simulink model "QCwithActDyn_NewPID"  (R2020a)
settings: Solver=FixedStepAuto  StartTime=0.0  StopTime=5+T  FixedStep=0.001  RelTol=1e-3
model workspace (MAT data in the model file):
  time_step = 0.01
values from neighbouring files (symbols this model uses):
  K_pitch = 30    [Parameters.m]
  K_roll = 30    [Parameters.m]
  K_z = 1.5059    [Parameters.m]    (also in descent2.m = 2)
  kD_P = 0.1529    [Parameters.m]
  kD_R = 0.1564    [Parameters.m]
  kD_x = 9.3766    [Parameters.m]
  kD_y = 9.54    [Parameters.m]
  kD_z = 17    [Parameters.m]    (also in descent2.m = 17.85; gradient_descent.m = 0.95*kD_z)
  kI_x = 0    [Parameters.m]
  kI_y = 0    [Parameters.m]
  kP_P = 1.3542    [Parameters.m]
  kP_R = 1.3852    [Parameters.m]
  kP_x = 34.159    [Parameters.m]
  kP_y = 34.775    [Parameters.m]
  kP_z = 40    [Parameters.m]    (also in descent2.m; gradient_descent.m = 0.95*kP_z)
  PVA = 1    [Parameters.m]
  T_aero = 1.5    [Parameters.m]    (also in descent2.m = 2)
  T_motor = 0.015    [Parameters.m]
  T_pitch = 0.2005    [Parameters.m]
  tau_pitch = 0.025    [Parameters.m]
  tau_roll = 0.025    [Parameters.m]
  tau_x = 0.0223    [Parameters.m]
  tau_y = 0.0223    [Parameters.m]
  tau_z = 0.027    [Parameters.m]
  X_Ch = 1    [Parameters.m]
  Y_Ch = 1    [Parameters.m]
libraries: simulink_extras x2
settings Model: Creator=Abdulaziz Y. Alkayas  LastModifiedBy=anees
settings SolverCC: SolverResetMethod=Robust
settings DebuggingCC: UnconnectedInputMsg=none  UnconnectedOutputMsg=none  ArithmeticOperatorsInVariantConditions=warning
settings HardwareCC: TargetBitPerPointer=64  TargetBitPerSizeT=64  TargetBitPerPtrDiffT=64  TargetLongLongMode=on  TargetIntDivRoundTo=Zero  TargetEndianess=LittleEndian  TargetWordSize=64  TargetHWDeviceType=MATLAB Host  ProdEqTarget=off
settings SFSimCC: CustomCodeUndefinedFunction=UseInterfaceOnly
settings RTWCC: Description=Generic Real-Time Target

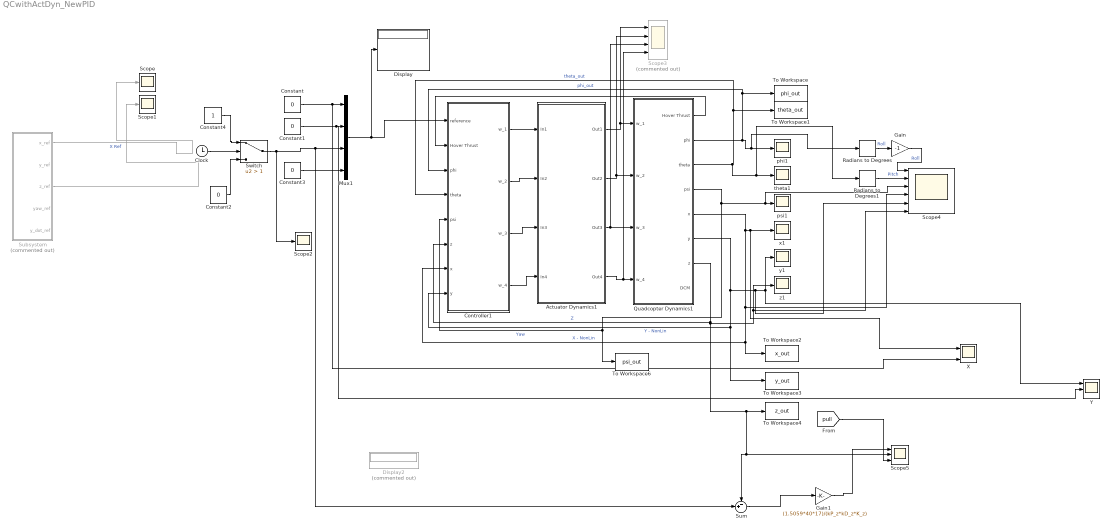
== system QCwithActDyn_NewPID ==
  Actuator Dynamics1 : Subsystem
  Clock : Clock
  Constant{,1..3} (4 alike) : Constant  Value=0
  Constant4 : Constant
  Controller1 : Subsystem
  Display : Display
  Display2 : Display  Commented=on
  Gain : Gain  Gain=-1
  Gain1 : Gain  Gain=(1.5059*40*17)/(kP_z*kD_z*K_z)
  Mux1 : Mux
  Quadcopter Dynamics1 : Subsystem
  Radians to Degrees : simulink_extras/Transformations/Radians to Degrees
  Radians to Degrees1 : simulink_extras/Transformations/Radians to Degrees
  Scope : Scope
  Scope1 : Scope
  Scope2 : Scope
  Scope3 : Scope  Commented=on  NumInputPorts=4
  Scope4 : Scope  NumInputPorts=6
  Scope5 : Scope  NumInputPorts=3
  Subsystem : Subsystem  Commented=on
  Sum : Sum  Inputs=-+|
  Switch : Switch  Criteria=u2 > Threshold  Threshold=1
  To Workspace : ToWorkspace  VariableName=phi_out  SaveFormat=Timeseries  SampleTime=-1
  To Workspace1 : ToWorkspace  VariableName=theta_out  SaveFormat=Timeseries  SampleTime=-1
  To Workspace2 : ToWorkspace  VariableName=x_out  SaveFormat=Timeseries  SampleTime=-1
  To Workspace3 : ToWorkspace  VariableName=y_out  SaveFormat=Timeseries  SampleTime=-1
  To Workspace4 : ToWorkspace  VariableName=z_out  SaveFormat=Timeseries  SampleTime=-1
  To Workspace6 : ToWorkspace  VariableName=psi_out  SaveFormat=Timeseries  SampleTime=-1
  X : Scope  NumInputPorts=3
  Y : Scope  NumInputPorts=3
  phi1 : Scope
  psi1 : Scope
  theta1 : Scope
  x1 : Scope
  y1 : Scope
  z1 : Scope
  wires:
  Controller1/4(w_4) -> Actuator Dynamics1/4(In4)
  Controller1/3(w_3) -> Actuator Dynamics1/3(In3)
  Controller1/2(w_2) -> Actuator Dynamics1/2(In2)
  Controller1/1(w_1) -> Actuator Dynamics1/1(In1)
  Quadcopter Dynamics1/4(psi) -> To Workspace6/1, Controller1/5(psi), psi1/1, Scope4/3  "Yaw"
  Quadcopter Dynamics1/7(z) -> Sum/1, Scope5/2, To Workspace4/1, z1/1, Scope4/6, Controller1/6(z)  "Z"
  Quadcopter Dynamics1/1(Hover Thrust) -> Controller1/2(Hover Thrust)
  Quadcopter Dynamics1/5(x) -> Scope4/4, To Workspace2/1, Controller1/7(x), X/1, x1/1  "X - NonLin"
  Quadcopter Dynamics1/6(y) -> To Workspace3/1, Controller1/8(y), Y/1, y1/1, Scope4/5  "Y - NonLin"
  Subsystem/3("z_ref ") -> Scope1/1
  Actuator Dynamics1/1(Out1) -> Scope3/1, Quadcopter Dynamics1/1(w_1)
  Actuator Dynamics1/2(Out2) -> Quadcopter Dynamics1/2(w_2), Scope3/2
  Actuator Dynamics1/3(Out3) -> Quadcopter Dynamics1/3(w_3), Scope3/3
  Actuator Dynamics1/4(Out4) -> Quadcopter Dynamics1/4(w_4), Scope3/4
  Radians to Degrees/1 -> Gain/1  "Roll"
  Radians to Degrees1/1 -> Scope4/2  "Pitch"
  Gain/1 -> Scope4/1  "Roll"
  Subsystem/1("x_ref ") -> Scope/1  "X Ref"
  Constant1/1 -> Y/2, Mux1/2
  Constant/1 -> X/3, Mux1/1
  Constant3/1 -> Mux1/4
  Mux1/1 -> Display/1, Controller1/1(reference)
  Quadcopter Dynamics1/2(phi) -> Controller1/3(phi), To Workspace/1, Radians to Degrees/1, phi1/1  "phi_out"
  Quadcopter Dynamics1/3(theta) -> Radians to Degrees1/1, theta1/1, Controller1/4(theta), To Workspace1/1  "theta_out"
  Constant2/1 -> Switch/3
  Switch/1 -> Sum/2, Mux1/3, Scope2/1
  Constant4/1 -> Switch/1
  Clock/1 -> Switch/2
  [pull] -> Scope5/3
  Gain1/1 -> Scope5/1
  Sum/1 -> Gain1/1

== system QCwithActDyn_NewPID/Actuator Dynamics1 ==
  In1 : Inport
  In2 : Inport  Port=2
  In3 : Inport  Port=3
  In4 : Inport  Port=4
  Transfer Fcn{1..4} (4 alike) : TransferFcn  Denominator=[T_motor 1]
  Out1 : Outport
  Out2 : Outport  Port=2
  Out3 : Outport  Port=3
  Out4 : Outport  Port=4
  wires:
  In4/1 -> Transfer Fcn2/1
  Transfer Fcn2/1 -> Out4/1
  Transfer Fcn1/1 -> Out3/1
  In2/1 -> Transfer Fcn4/1
  Transfer Fcn4/1 -> Out2/1
  Transfer Fcn3/1 -> Out1/1
  In3/1 -> Transfer Fcn1/1
  In1/1 -> Transfer Fcn3/1

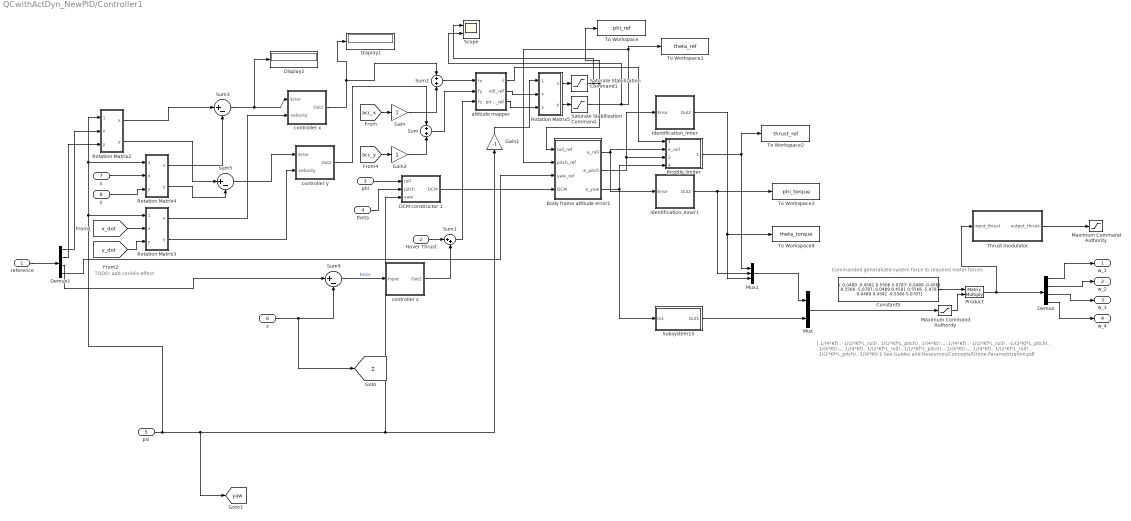
== system QCwithActDyn_NewPID/Controller1 ==
  note: TODO: add coriolis effect
  note: [ 1/(4*Kf) , -1/(2*Kf*L_roll) , 1/(2*Kf*L_pitch) , 1/(4*Kt) ;...
      | 1/(4*Kf) , -1/(2*Kf*L_roll) , -1/(2*Kf*L_pitch) , -1/(4*Kt) ;...
      | 1/(4*Kf) , 1/(2*Kf*L_roll) , 1/(2*Kf*L_pitch) , -1/(4*Kt) ;...
      | 1/(4*Kf) , 1/(2*Kf*L_roll) , -1/(2*Kf*L_pitch) , 1/(4*Kt) ];
      |
      | See Guides and Resources/Concepts/Drone Parametrization.pdf
  note: Commanded generalized system force to required motor forces
  reference : Inport
  Hover Thrust : Inport  Port=2
  phi : Inport  Port=3
  theta : Inport  Port=4
  psi : Inport  Port=5
  z : Inport  Port=6
  x : Inport  Port=7
  y : Inport  Port=8
  Body frame attitude error1 : MATLAB Function  TreatAsAtomicUnit=on
  Constant5 : Constant  Value=|
      | [ 0.0489   -0.4581    0.5566    5.0787;
      |   0.0489   -0.4581   -0.5566   -5.0787;
      |   0.0489    0.4581    0.5566   -5.0787;
      |   0.0489    0.4581   -0.5566    5.0787]
  DCM constructor 1 : MATLAB Function  TreatAsAtomicUnit=on
  Demux : Demux
  Demux1 : Demux
  Display1 : Display
  Display2 : Display
  Gain : Gain
  Gain1 : Gain  Gain=-1
  Gain2 : Gain
  Identification_Inner : Subsystem
  Identification_Inner1 : Subsystem
  Maximum Command Authority : Saturate  UpperLimit=[Inf Inf Inf Inf]  LowerLimit=[-inf -Inf -Inf -Inf]
  "Maximum Command Authority " : Saturate  UpperLimit=[1 1 1 1]  LowerLimit=[0 0 0 0]
  Mux : Mux  Inputs=[3, 1]
  Mux1 : Mux  Inputs=3
  Product : Product  Multiplication=Matrix(*)
  Rotation Matrix2 : Subsystem
  Rotation Matrix3 : Subsystem
  Rotation Matrix4 : Subsystem
  Rotation Matrix5 : Subsystem
  Saturate Stabilization Command : Saturate  UpperLimit=pi/2  LowerLimit=-pi/2
  Saturate Stabilization Command1 : Saturate  UpperLimit=pi/2  LowerLimit=-pi/2
  Scope : Scope  NumInputPorts=2
  Subsystem15 : Subsystem
  Sum : Sum
  Sum1 : Sum  Inputs=|++
  Sum2 : Sum
  Sum3 : Sum  Inputs=|+-
  Sum5 : Sum  Inputs=|+-
  Sum9 : Sum  Inputs=|+-
  Thrust modulator : MATLAB Function  TreatAsAtomicUnit=on
  To Workspace : ToWorkspace  VariableName=phi_ref  SaveFormat=Structure With Time  SampleTime=-1
  To Workspace1 : ToWorkspace  VariableName=theta_ref  SaveFormat=Structure With Time  SampleTime=-1
  To Workspace2 : ToWorkspace  VariableName=thrust_ref  SaveFormat=Timeseries  SampleTime=-1
  To Workspace3 : ToWorkspace  VariableName=phi_torque  SaveFormat=Timeseries  SampleTime=-1
  To Workspace4 : ToWorkspace  VariableName=theta_torque  SaveFormat=Timeseries  SampleTime=-1
  "attitude mapper " : MATLAB Function  TreatAsAtomicUnit=on
  controller x : Subsystem
  controller y : Subsystem
  controller z : Subsystem
  throttle limiter : MATLAB Function  TreatAsAtomicUnit=on
  w_1 : Outport
  w_2 : Outport  Port=2
  w_3 : Outport  Port=3
  w_4 : Outport  Port=4
  tag scope: yaw=global, z=global
  wires:
  z/1 -> Sum9/2, [z]
  Maximum Command Authority/1 -> Product/2
  Mux/1 -> Maximum Command Authority/1
  Constant5/1 -> Product/1
  Demux/2 -> w_2/1
  Demux/3 -> w_3/1
  Demux/4 -> w_4/1
  Sum3/1 -> Display2/1, controller x/1(Error)
  Sum5/1 -> controller y/1(Error)
  Hover Thrust/1 -> Sum1/1
  Demux/1 -> w_1/1
  Sum9/1 -> controller z/1(Input)  "Error"
  controller z/1(Out2) -> Sum1/2
  reference/1 -> Demux1/1
  Demux1/3 -> Sum9/1
  controller x/1(Out2) -> Display1/1, Sum2/1
  controller y/1(Out2) -> Sum/1
  Sum1/1 -> "attitude mapper "/3(fz)
  Demux1/4 -> Body frame attitude error1/3(yaw_ref)
  Body frame attitude error1/3(e_yaw) -> throttle limiter/4(e_yaw), Subsystem15/1(In1)
  Body frame attitude error1/2(e_pitch) -> Identification_Inner/1(Error), throttle limiter/3(e_pitch)
  Body frame attitude error1/1(e_roll) -> Identification_Inner1/1(Error), throttle limiter/2(e_roll)
  Demux1/1 -> Rotation Matrix2/2("x ")
  Demux1/2 -> Rotation Matrix2/3(y)
  Rotation Matrix2/1(x) -> Sum3/1
  Rotation Matrix2/2("y ") -> Sum5/1
  [x_dot] -> Rotation Matrix3/2("x ")
  [y_dot] -> Rotation Matrix3/3(y)
  Rotation Matrix3/1(x) -> controller x/2("velocity ")
  Rotation Matrix3/2("y ") -> controller y/2("velocity ")
  x/1 -> Rotation Matrix4/2("x ")
  y/1 -> Rotation Matrix4/3(y)
  Rotation Matrix4/1(x) -> Sum3/2
  Rotation Matrix4/2("y ") -> Sum5/2
  DCM constructor 1/1(DCM) -> Body frame attitude error1/4(DCM)
  "attitude mapper "/2(roll_ref) -> Rotation Matrix5/2("x ")
  "attitude mapper "/3(pitch_ref) -> Rotation Matrix5/3(y)
  Rotation Matrix5/1(x) -> Saturate Stabilization Command1/1
  Identification_Inner1/1(Out2) -> Mux1/2, To Workspace3/1
  Identification_Inner/1(Out2) -> Mux1/3, To Workspace4/1
  Mux1/1 -> Mux/1
  psi/1 -> Rotation Matrix4/1("yaw "), Rotation Matrix2/1("yaw "), Rotation Matrix3/1("yaw "), [yaw], Gain1/1, DCM constructor 1/3(yaw)
  Gain1/1 -> Rotation Matrix5/1("yaw ")
  Rotation Matrix5/2("y ") -> Saturate Stabilization Command/1
  Saturate Stabilization Command/1 -> Scope/2, To Workspace1/1, Body frame attitude error1/2(pitch_ref)
  Saturate Stabilization Command1/1 -> Scope/1, To Workspace/1, Body frame attitude error1/1(roll_ref)
  phi/1 -> DCM constructor 1/1(roll)
  theta/1 -> DCM constructor 1/2(pitch)
  "attitude mapper "/1(f) -> throttle limiter/1(throttle_in)
  throttle limiter/1(throttle_out) -> Mux1/1, To Workspace2/1
  Product/1 -> Thrust modulator/1(input_thrust), Demux/1
  Thrust modulator/1(output_thrust) -> "Maximum Command Authority "/1
  Sum2/1 -> "attitude mapper "/1(fx)
  Sum/1 -> "attitude mapper "/2(fy)
  [acc_x] -> Gain/1
  [acc_y] -> Gain2/1
  Subsystem15/1(Out1) -> Mux/2
  Gain/1 -> Sum2/2
  Gain2/1 -> Sum/2

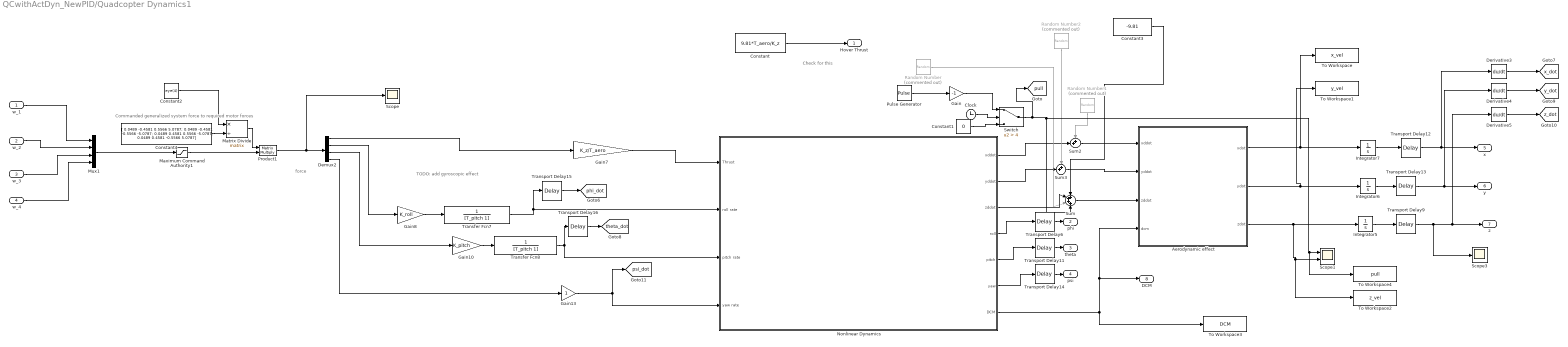
== system QCwithActDyn_NewPID/Quadcopter Dynamics1 ==
  note: force
  note: TODO: add gyroscopic effect
  note: Check for this
  note: Commanded generalized system force to required motor forces
  w_1 : Inport
  w_2 : Inport  Port=2
  w_3 : Inport  Port=3
  w_4 : Inport  Port=4
  "Aerodynamic effect " : Subsystem
  Clock : Clock
  Constant : Constant  Value=9.81*T_aero/K_z
  Constant1 : Constant  Value=0
  Constant2 : Constant  Value=eye(4)
  Constant3 : Constant  Value=-9.81
  Constant4 : Constant  Value=|
      | [ 0.0489   -0.4581    0.5566    5.0787;
      |   0.0489   -0.4581   -0.5566   -5.0787;
      |   0.0489    0.4581    0.5566   -5.0787;
      |   0.0489    0.4581   -0.5566    5.0787]
  Demux2 : Demux
  Derivative3 : Derivative
  Derivative4 : Derivative
  Derivative5 : Derivative
  Gain : Gain  Gain=-1
  Gain10 : Gain  Gain=K_pitch
  Gain13 : Gain
  Gain7 : Gain  Gain=K_z/T_aero
  Gain8 : Gain  Gain=K_roll
  Integrator5 : Integrator
  Integrator6 : Integrator
  Integrator7 : Integrator
  Matrix Divide : Product  Inputs=*/  Multiplication=Matrix(*)
  Maximum Command Authority1 : Saturate  UpperLimit=[Inf Inf Inf Inf]  LowerLimit=[-Inf -Inf -Inf -Inf]
  Mux1 : Mux
  Nonlinear Dynamics : Subsystem
  Product1 : Product  Multiplication=Matrix(*)
  Pulse Generator : DiscretePulseGenerator  PulseType=Time based  Amplitude=5  Period=10  PulseWidth=5
  Random Number : RandomNumber  Commented=on  SampleTime=0.01
  Random Number1 : RandomNumber  Commented=on  SampleTime=0.01
  Random Number2 : RandomNumber  Commented=on  SampleTime=0.01
  Scope : Scope
  Scope1 : Scope  NumInputPorts=2
  Scope3 : Scope
  Sum : Sum  Inputs=++++
  Sum2 : Sum  Inputs=++|
  Sum3 : Sum  Inputs=++|
  Switch : Switch  Criteria=u2 > Threshold  Threshold=4
  To Workspace : ToWorkspace  VariableName=x_vel  SaveFormat=Structure With Time  SampleTime=-1
  To Workspace1 : ToWorkspace  VariableName=y_vel  SaveFormat=Structure With Time  SampleTime=-1
  To Workspace2 : ToWorkspace  VariableName=z_vel  SaveFormat=Timeseries  SampleTime=-1
  To Workspace3 : ToWorkspace  VariableName=DCM  SaveFormat=Timeseries  SampleTime=-1
  To Workspace4 : ToWorkspace  VariableName=pull  SaveFormat=Timeseries  SampleTime=-1
  Transfer Fcn7 : TransferFcn  Denominator=[T_pitch 1]
  Transfer Fcn8 : TransferFcn  Denominator=[T_pitch 1]
  Transport Delay11 : TransportDelay  DelayTime=tau_pitch
  Transport Delay12 : TransportDelay  DelayTime=tau_x
  Transport Delay13 : TransportDelay  DelayTime=tau_y
  Transport Delay14 : TransportDelay  DelayTime=0
  Transport Delay15 : TransportDelay  DelayTime=tau_roll
  Transport Delay16 : TransportDelay  DelayTime=tau_pitch
  Transport Delay6 : TransportDelay  DelayTime=tau_roll
  Transport Delay9 : TransportDelay  DelayTime=tau_z
  Hover Thrust : Outport
  phi : Outport  Port=2
  theta : Outport  Port=3
  psi : Outport  Port=4
  x : Outport  Port=5
  y : Outport  Port=6
  z : Outport  Port=7
  DCM : Outport  Port=8
  tag scope: phi_dot=global, psi_dot=global, pull=global, theta_dot=global, x_dot=global, y_dot=global, z_dot=global
  wires:
  w_2/1 -> Mux1/2
  w_3/1 -> Mux1/3
  w_4/1 -> Mux1/4
  Maximum Command Authority1/1 -> Product1/2
  Constant2/1 -> Matrix Divide/1
  Mux1/1 -> Maximum Command Authority1/1
  Constant4/1 -> Matrix Divide/2
  w_1/1 -> Mux1/1
  Nonlinear Dynamics/7(DCM) -> "Aerodynamic effect "/4(dcm), DCM/1, To Workspace3/1
  Integrator7/1 -> Transport Delay12/1
  Demux2/4 -> Gain13/1
  Demux2/3 -> Gain10/1
  Demux2/2 -> Gain8/1
  Transfer Fcn8/1 -> Transport Delay16/1, Nonlinear Dynamics/3(pitch rate)
  Gain10/1 -> Transfer Fcn8/1
  Gain8/1 -> Transfer Fcn7/1
  Nonlinear Dynamics/4(roll) -> Transport Delay6/1
  Nonlinear Dynamics/5("pitch ") -> Transport Delay11/1
  Sum/1 -> "Aerodynamic effect "/3(zddot)
  Transport Delay11/1 -> theta/1
  Transport Delay6/1 -> phi/1
  Integrator5/1 -> Transport Delay9/1
  Transport Delay12/1 -> Derivative3/1, x/1
  Integrator6/1 -> Transport Delay13/1
  Transfer Fcn7/1 -> Transport Delay15/1, Nonlinear Dynamics/2("roll rate ")
  "Aerodynamic effect "/3(zdot) -> Scope1/2, To Workspace2/1, Integrator5/1
  Constant3/1 -> Sum/1
  Constant/1 -> Hover Thrust/1
  Demux2/1 -> Gain7/1
  Transport Delay14/1 -> psi/1
  Nonlinear Dynamics/6(yaw) -> Transport Delay14/1
  Transport Delay15/1 -> [phi_dot]
  Transport Delay16/1 -> [theta_dot]
  Gain13/1 -> [psi_dot], Nonlinear Dynamics/4("yaw rate ")
  Derivative5/1 -> [z_dot]
  Derivative4/1 -> [y_dot]
  Transport Delay9/1 -> Scope3/1, Derivative5/1, z/1
  Derivative3/1 -> [x_dot]
  Transport Delay13/1 -> Derivative4/1, y/1
  Product1/1 -> Demux2/1, Scope/1
  Matrix Divide/1 -> Product1/1
  "Aerodynamic effect "/2(ydot) -> To Workspace1/1, Integrator6/1
  "Aerodynamic effect "/1("xdot ") -> To Workspace/1, Integrator7/1
  Gain7/1 -> Nonlinear Dynamics/1(Thrust)
  Nonlinear Dynamics/1(xddot) -> Sum2/2
  Sum2/1 -> "Aerodynamic effect "/1(xddot)
  Nonlinear Dynamics/2(yddot) -> Sum3/2
  Sum3/1 -> "Aerodynamic effect "/2(yddot)
  Random Number/1 -> Sum/3
  Random Number2/1 -> Sum3/1
  Random Number1/1 -> Sum2/1
  Pulse Generator/1 -> Gain/1
  Gain/1 -> Switch/1
  Nonlinear Dynamics/3(zddot) -> Sum/2
  Clock/1 -> Switch/2
  Switch/1 -> [pull], Sum/4, To Workspace4/1, Scope1/1
  Constant1/1 -> Switch/3

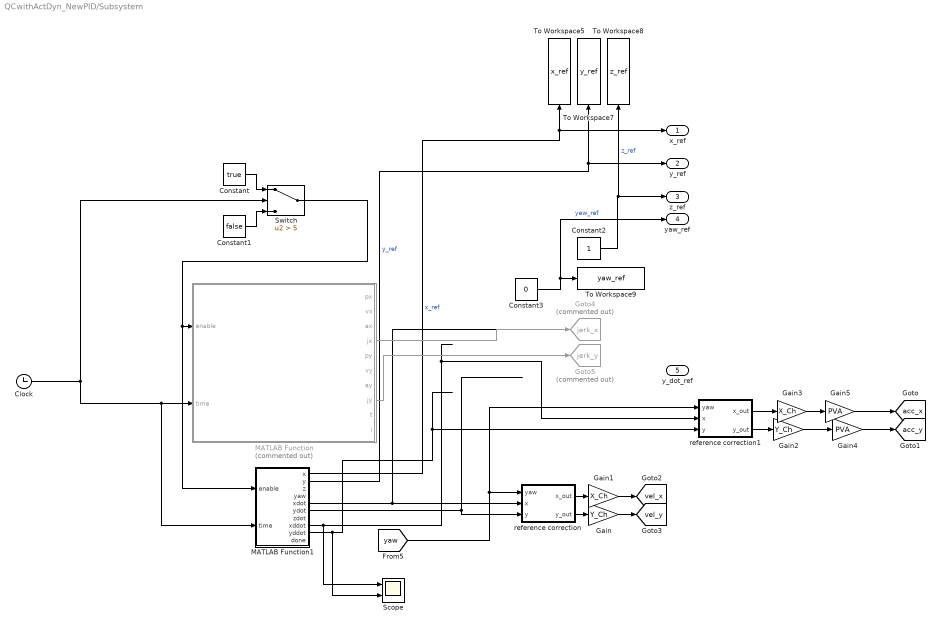
== system QCwithActDyn_NewPID/Subsystem ==
  Clock : Clock
  Constant : Constant  Value=true
  Constant1 : Constant  Value=false
  Constant2 : Constant
  Constant3 : Constant  Value=0
  Gain : Gain  Gain=Y_Ch
  Gain1 : Gain  Gain=X_Ch
  Gain2 : Gain  Gain=Y_Ch
  Gain3 : Gain  Gain=X_Ch
  Gain4 : Gain  Gain=PVA
  Gain5 : Gain  Gain=PVA
  Goto4 : Goto  Commented=on  GotoTag=jerk_x  TagVisibility=global
  Goto5 : Goto  Commented=on  GotoTag=jerk_y  TagVisibility=global
  MATLAB Function : MATLAB Function  Commented=on  TreatAsAtomicUnit=on
  MATLAB Function1 : MATLAB Function  TreatAsAtomicUnit=on
  Scope : Scope  NumInputPorts=2
  Switch : Switch  Criteria=u2 > Threshold  Threshold=5
  To Workspace5 : ToWorkspace  VariableName=x_ref  SaveFormat=Timeseries  SampleTime=-1
  To Workspace7 : ToWorkspace  VariableName=y_ref  SaveFormat=Timeseries  SampleTime=-1
  To Workspace8 : ToWorkspace  VariableName=z_ref  SaveFormat=Timeseries  SampleTime=-1
  To Workspace9 : ToWorkspace  VariableName=yaw_ref  SaveFormat=Timeseries  SampleTime=-1
  reference correction : MATLAB Function  TreatAsAtomicUnit=on
  reference correction1 : MATLAB Function  TreatAsAtomicUnit=on
  "x_ref " : Outport
  "y_ref " : Outport  Port=2
  "z_ref " : Outport  Port=3
  "yaw_ref " : Outport  Port=4
  "y_dot_ref " : Outport  Port=5
  tag scope: acc_x=global, acc_y=global, vel_x=global, vel_y=global
  wires:
  Switch/1 -> MATLAB Function1/1(enable), MATLAB Function/1(enable)
  Clock/1 -> Switch/2, MATLAB Function1/2(time), MATLAB Function/2(time)
  Constant2/1 -> To Workspace8/1, "z_ref "/1  "z_ref"
  MATLAB Function1/1(x) -> "x_ref "/1, To Workspace5/1  "x_ref"
  MATLAB Function1/2(y) -> "y_ref "/1, To Workspace7/1  "y_ref"
  Constant3/1 -> "yaw_ref "/1, To Workspace9/1  "yew_ref"
  Constant/1 -> Switch/1
  Constant1/1 -> Switch/3
  MATLAB Function1/8(xddot) -> Scope/1, reference correction1/2(x)
  MATLAB Function1/9(yddot) -> Scope/2, reference correction1/3(y)
  MATLAB Function1/5(xdot) -> reference correction/2(x)
  MATLAB Function1/6(ydot) -> reference correction/3(y)
  MATLAB Function/4(jx) -> Goto4/1
  MATLAB Function/8(jy) -> Goto5/1
  reference correction/2(y_out) -> Gain/1
  reference correction/1(x_out) -> Gain1/1
  [yaw] -> reference correction1/1(yaw), reference correction/1(yaw)
  Gain/1 -> [vel_y]
  Gain1/1 -> [vel_x]
  reference correction1/1(x_out) -> Gain3/1
  reference correction1/2(y_out) -> Gain2/1
  Gain3/1 -> Gain5/1
  Gain2/1 -> Gain4/1
  Gain5/1 -> [acc_x]
  Gain4/1 -> [acc_y]

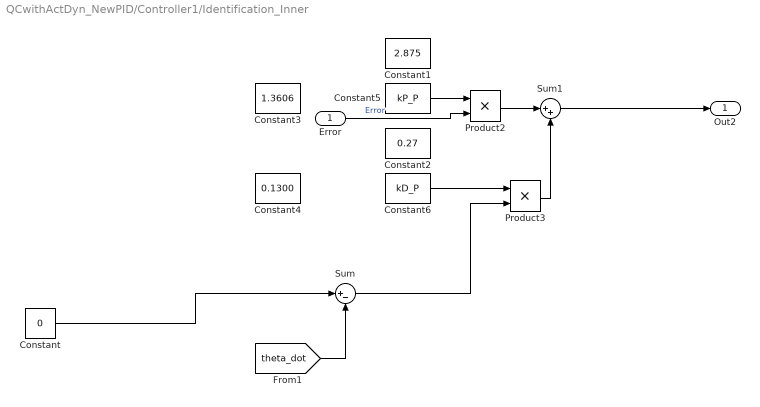
== system QCwithActDyn_NewPID/Controller1/Identification_Inner ==
  Error : Inport
  Constant : Constant  Value=0
  Constant1 : Constant  Value=2.875
  Constant2 : Constant  Value=0.27
  Constant3 : Constant  Value=1.3606
  Constant4 : Constant  Value=0.1300
  Constant5 : Constant  Value=kP_P
  Constant6 : Constant  Value=kD_P
  Product2 : Product
  Product3 : Product
  Sum : Sum  Inputs=|+-
  Sum1 : Sum  Inputs=|++
  Out2 : Outport
  wires:
  Error/1 -> Product2/2  "Error"
  [theta_dot] -> Sum/2
  Product2/1 -> Sum1/1
  Constant6/1 -> Product3/1
  Sum/1 -> Product3/2
  Constant5/1 -> Product2/1
  Sum1/1 -> Out2/1
  Product3/1 -> Sum1/2
  Constant/1 -> Sum/1

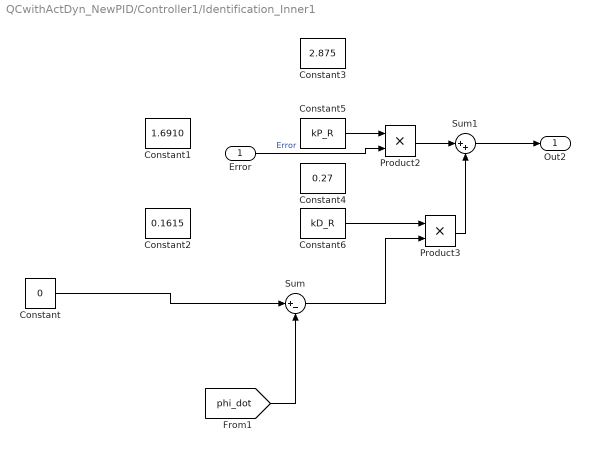
== system QCwithActDyn_NewPID/Controller1/Identification_Inner1 ==
  Error : Inport
  Constant : Constant  Value=0
  Constant1 : Constant  Value=1.6910
  Constant2 : Constant  Value=0.1615
  Constant3 : Constant  Value=2.875
  Constant4 : Constant  Value=0.27
  Constant5 : Constant  Value=kP_R
  Constant6 : Constant  Value=kD_R
  Product2 : Product
  Product3 : Product
  Sum : Sum  Inputs=|+-
  Sum1 : Sum  Inputs=|++
  Out2 : Outport
  wires:
  Sum1/1 -> Out2/1
  Product3/1 -> Sum1/2
  Constant6/1 -> Product3/1
  Constant5/1 -> Product2/1
  [phi_dot] -> Sum/2
  Sum/1 -> Product3/2
  Product2/1 -> Sum1/1
  Error/1 -> Product2/2  "Error"
  Constant/1 -> Sum/1

== system QCwithActDyn_NewPID/Controller1/Rotation Matrix2 ==
  "yaw " : Inport
  "x " : Inport  Port=2
  y : Inport  Port=3
  reference correction : MATLAB Function  TreatAsAtomicUnit=on
  x : Outport
  "y " : Outport  Port=2
  wires:
  "yaw "/1 -> reference correction/1(yaw)
  "x "/1 -> reference correction/2(x)
  y/1 -> reference correction/3(y)
  reference correction/1(x_out) -> x/1
  reference correction/2(y_out) -> "y "/1

== system QCwithActDyn_NewPID/Controller1/Rotation Matrix3 ==
  "yaw " : Inport
  "x " : Inport  Port=2
  y : Inport  Port=3
  reference correction : MATLAB Function  TreatAsAtomicUnit=on
  x : Outport
  "y " : Outport  Port=2
  wires:
  reference correction/2(y_out) -> "y "/1
  reference correction/1(x_out) -> x/1
  y/1 -> reference correction/3(y)
  "x "/1 -> reference correction/2(x)
  "yaw "/1 -> reference correction/1(yaw)

== system QCwithActDyn_NewPID/Controller1/Rotation Matrix4 ==
  "yaw " : Inport
  "x " : Inport  Port=2
  y : Inport  Port=3
  reference correction : MATLAB Function  TreatAsAtomicUnit=on
  x : Outport
  "y " : Outport  Port=2
  wires:
  "yaw "/1 -> reference correction/1(yaw)
  "x "/1 -> reference correction/2(x)
  y/1 -> reference correction/3(y)
  reference correction/1(x_out) -> x/1
  reference correction/2(y_out) -> "y "/1

== system QCwithActDyn_NewPID/Controller1/Rotation Matrix5 ==
  "yaw " : Inport
  "x " : Inport  Port=2
  y : Inport  Port=3
  reference correction : MATLAB Function  TreatAsAtomicUnit=on
  x : Outport
  "y " : Outport  Port=2
  wires:
  "yaw "/1 -> reference correction/1(yaw)
  "x "/1 -> reference correction/2(x)
  y/1 -> reference correction/3(y)
  reference correction/1(x_out) -> x/1
  reference correction/2(y_out) -> "y "/1

== system QCwithActDyn_NewPID/Controller1/Subsystem15 ==
  In1 : Inport
  Gain2 : Gain  Gain=5
  Gain3 : Gain  Gain=5
  Sum6 : Sum  Inputs=|-+
  Out1 : Outport
  wires:
  Gain3/1 -> Sum6/2
  Gain2/1 -> Sum6/1
  Sum6/1 -> Out1/1
  In1/1 -> Gain3/1
  [psi_dot] -> Gain2/1

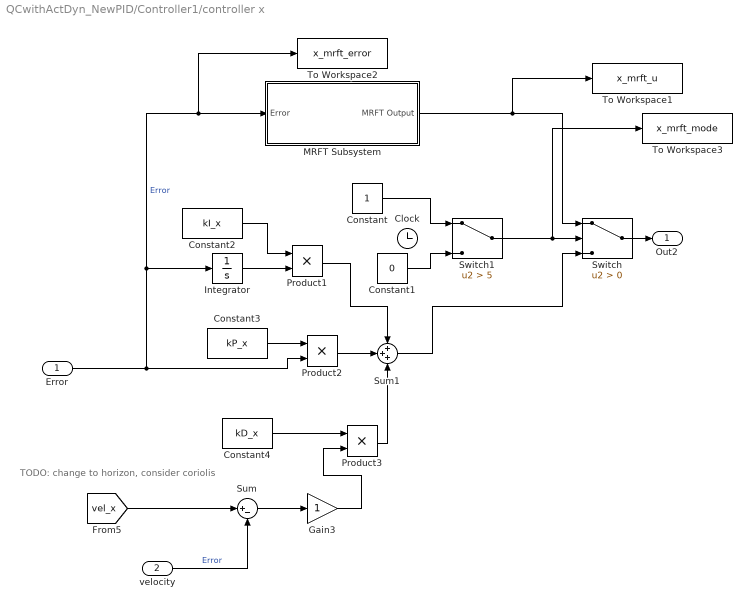
== system QCwithActDyn_NewPID/Controller1/controller x ==
  note: TODO: change to horizon, consider coriolis
  Error : Inport
  "velocity " : Inport  Port=2
  Clock : Clock
  Constant : Constant
  Constant1 : Constant  Value=0
  Constant2 : Constant  Value=kI_x
  Constant3 : Constant  Value=kP_x
  Constant4 : Constant  Value=kD_x
  Gain3 : Gain
  Integrator : Integrator
  MRFT Subsystem : Subsystem
  Product1 : Product
  Product2 : Product
  Product3 : Product
  Sum : Sum  Inputs=|+-
  Sum1 : Sum  Inputs=+++
  Switch : Switch  Criteria=u2 > Threshold
  Switch1 : Switch  Criteria=u2 > Threshold  Threshold=5
  To Workspace1 : ToWorkspace  VariableName=x_mrft_u  SaveFormat=Timeseries  SampleTime=0.001
  To Workspace2 : ToWorkspace  VariableName=x_mrft_error  SaveFormat=Timeseries  SampleTime=0.001
  To Workspace3 : ToWorkspace  VariableName=x_mrft_mode  SaveFormat=Timeseries  SampleTime=0.001
  Out2 : Outport
  wires:
  Error/1 -> Integrator/1, To Workspace2/1, MRFT Subsystem/1(Error), Product2/2  "Error"
  Constant4/1 -> Product3/1
  Gain3/1 -> Product3/2
  Constant3/1 -> Product2/1
  Constant1/1 -> Switch1/3
  Constant/1 -> Switch1/1
  MRFT Subsystem/1(MRFT Output) -> To Workspace1/1, Switch/1
  Switch1/1 -> To Workspace3/1, Switch/2
  Sum1/1 -> Switch/3
  Switch/1 -> Out2/1
  "velocity "/1 -> Sum/2  "Error"
  Integrator/1 -> Product1/2
  Constant2/1 -> Product1/1
  Product1/1 -> Sum1/1
  Product3/1 -> Sum1/3
  Product2/1 -> Sum1/2
  Sum/1 -> Gain3/1
  [vel_x] -> Sum/1

== system QCwithActDyn_NewPID/Controller1/controller y ==
  Error : Inport
  "velocity " : Inport  Port=2
  Constant1 : Constant  Value=kI_y
  Constant3 : Constant  Value=kP_y
  Constant4 : Constant  Value=kD_y
  Integrator : Integrator
  Product1 : Product
  Product2 : Product
  Product3 : Product
  Sum : Sum  Inputs=|+-
  Sum1 : Sum  Inputs=+++
  Out2 : Outport
  wires:
  Constant4/1 -> Product3/1
  Sum/1 -> Product3/2
  Constant3/1 -> Product2/1
  Sum1/1 -> Out2/1
  Error/1 -> Integrator/1, Product2/2  "Error"
  Product3/1 -> Sum1/3
  Product2/1 -> Sum1/2
  Integrator/1 -> Product1/2
  Constant1/1 -> Product1/1
  Product1/1 -> Sum1/1
  "velocity "/1 -> Sum/2  "Error"
  [vel_y] -> Sum/1

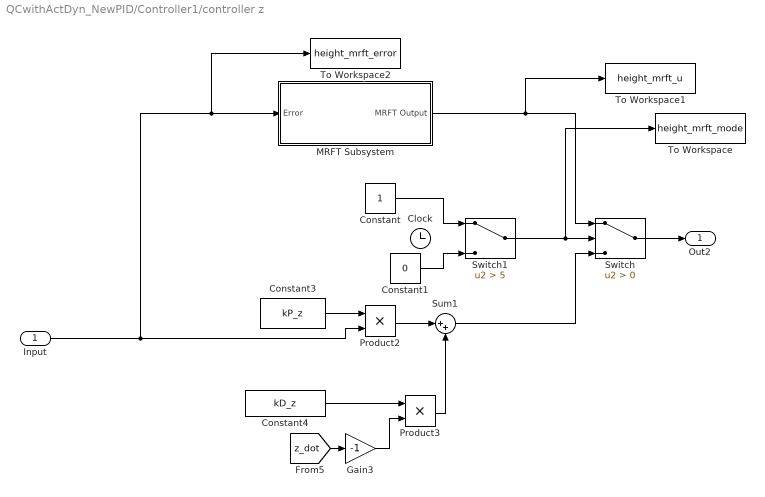
== system QCwithActDyn_NewPID/Controller1/controller z ==
  Input : Inport
  Clock : Clock
  Constant : Constant
  Constant1 : Constant  Value=0
  Constant3 : Constant  Value=kP_z
  Constant4 : Constant  Value=kD_z
  Gain3 : Gain  Gain=-1
  MRFT Subsystem : Subsystem
  Product2 : Product
  Product3 : Product
  Sum1 : Sum  Inputs=|++
  Switch : Switch  Criteria=u2 > Threshold
  Switch1 : Switch  Criteria=u2 > Threshold  Threshold=5
  To Workspace : ToWorkspace  VariableName=height_mrft_mode  SaveFormat=Timeseries  SampleTime=0.001
  To Workspace1 : ToWorkspace  VariableName=height_mrft_u  SaveFormat=Timeseries  SampleTime=0.001
  To Workspace2 : ToWorkspace  VariableName=height_mrft_error  SaveFormat=Timeseries  SampleTime=0.001
  Out2 : Outport
  wires:
  Constant4/1 -> Product3/1
  Gain3/1 -> Product3/2
  Product3/1 -> Sum1/2
  [z_dot] -> Gain3/1
  Product2/1 -> Sum1/1
  Constant3/1 -> Product2/1
  Input/1 -> To Workspace2/1, MRFT Subsystem/1(Error), Product2/2
  Switch/1 -> Out2/1
  Switch1/1 -> To Workspace/1, Switch/2
  Sum1/1 -> Switch/3
  MRFT Subsystem/1(MRFT Output) -> To Workspace1/1, Switch/1
  Constant1/1 -> Switch1/3
  Constant/1 -> Switch1/1

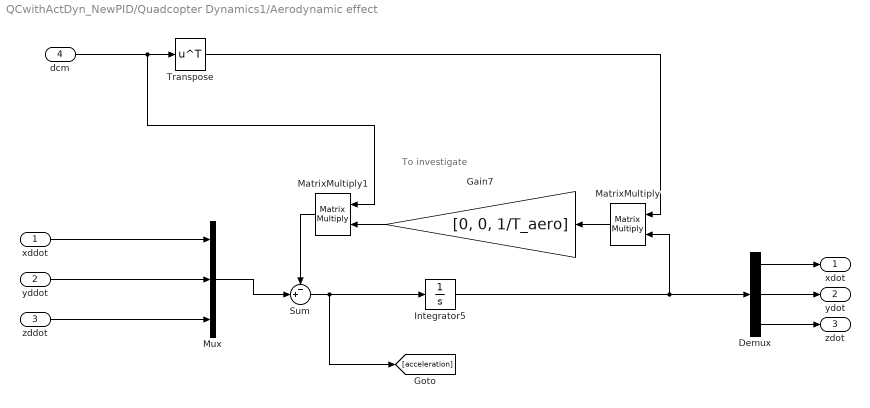
== system QCwithActDyn_NewPID/Quadcopter Dynamics1/Aerodynamic effect  ==
  note: To investigate
  xddot : Inport
  yddot : Inport  Port=2
  zddot : Inport  Port=3
  dcm : Inport  Port=4
  Demux : Demux  Outputs=3
  Gain7 : Gain  Gain=[0, 0, 1/T_aero]
  Integrator5 : Integrator
  MatrixMultiply : Product  Multiplication=Matrix(*)
  MatrixMultiply1 : Product  Multiplication=Matrix(*)
  Mux : Mux  Inputs=3
  Sum : Sum  Inputs=-+|
  Transpose : Math  Operator=transpose  SaturateOnIntegerOverflow=on
  "xdot " : Outport
  ydot : Outport  Port=2
  zdot : Outport  Port=3
  wires:
  Mux/1 -> Sum/2
  zddot/1 -> Mux/3
  MatrixMultiply/1 -> Gain7/1
  yddot/1 -> Mux/2
  xddot/1 -> Mux/1
  Demux/1 -> "xdot "/1
  Demux/2 -> ydot/1
  Demux/3 -> zdot/1
  Integrator5/1 -> MatrixMultiply/2, Demux/1
  Gain7/1 -> MatrixMultiply1/2
  Transpose/1 -> MatrixMultiply/1
  dcm/1 -> MatrixMultiply1/1, Transpose/1
  Sum/1 -> [acceleration], Integrator5/1
  MatrixMultiply1/1 -> Sum/1

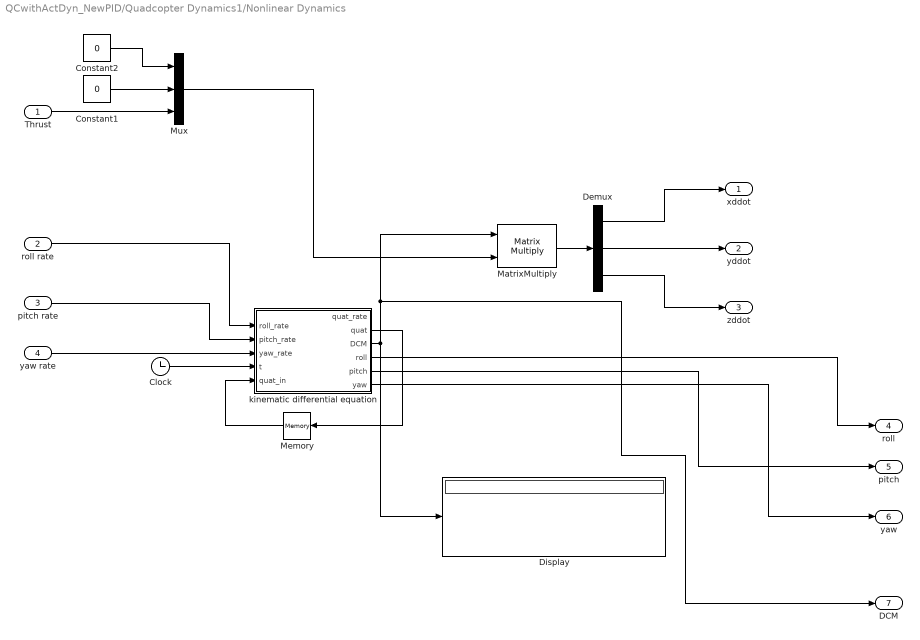
== system QCwithActDyn_NewPID/Quadcopter Dynamics1/Nonlinear Dynamics ==
  Thrust : Inport
  "roll rate " : Inport  Port=2
  pitch rate : Inport  Port=3
  "yaw rate " : Inport  Port=4
  Clock : Clock
  Constant1 : Constant  Value=0
  Constant2 : Constant  Value=0
  Demux : Demux  Outputs=3
  Display : Display
  MatrixMultiply : Product  Multiplication=Matrix(*)
  Memory : Memory  InitialCondition=[1 0 0 0]
  Mux : Mux  Inputs=3
  kinematic differential equation : MATLAB Function  TreatAsAtomicUnit=on
  xddot : Outport
  yddot : Outport  Port=2
  zddot : Outport  Port=3
  roll : Outport  Port=4
  "pitch " : Outport  Port=5
  yaw : Outport  Port=6
  DCM : Outport  Port=7
  wires:
  "yaw rate "/1 -> kinematic differential equation/3(yaw_rate)
  Thrust/1 -> Mux/3
  Constant2/1 -> Mux/1
  Constant1/1 -> Mux/2
  Mux/1 -> MatrixMultiply/2
  MatrixMultiply/1 -> Demux/1
  Demux/1 -> xddot/1
  Demux/2 -> yddot/1
  Demux/3 -> zddot/1
  "roll rate "/1 -> kinematic differential equation/1(roll_rate)
  pitch rate/1 -> kinematic differential equation/2(pitch_rate)
  Clock/1 -> kinematic differential equation/4(t)
  Memory/1 -> kinematic differential equation/5(quat_in)
  kinematic differential equation/5(pitch) -> "pitch "/1
  kinematic differential equation/4(roll) -> roll/1
  kinematic differential equation/2(quat) -> Memory/1
  kinematic differential equation/3(DCM) -> Display/1, DCM/1, MatrixMultiply/1
  kinematic differential equation/6(yaw) -> yaw/1

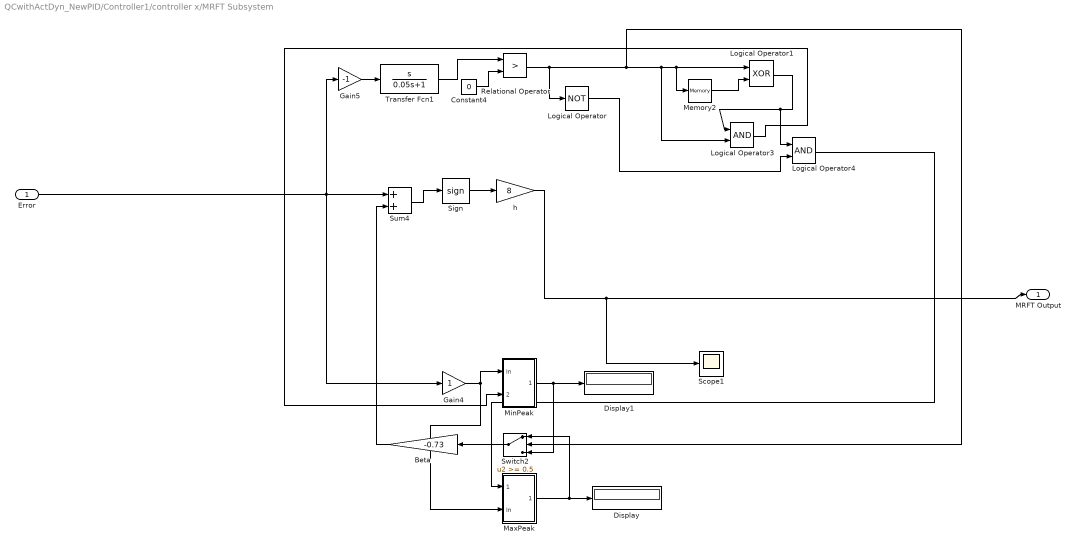
== system QCwithActDyn_NewPID/Controller1/controller x/MRFT Subsystem ==
  Error : Inport
  Beta : Gain  Gain=-0.73  SaturateOnIntegerOverflow=on  OutDataTypeStr=Inherit: Same as input  ParamDataTypeStr=Inherit: Same as input
  Constant4 : Constant  Value=0
  Display : Display
  Display1 : Display
  Gain4 : Gain  SaturateOnIntegerOverflow=on  OutDataTypeStr=Inherit: Same as input  ParamDataTypeStr=Inherit: Same as input
  Gain5 : Gain  Gain=-1  SaturateOnIntegerOverflow=on  OutDataTypeStr=Inherit: Same as input  ParamDataTypeStr=Inherit: Same as input
  Logical Operator : Logic  Operator=NOT  Inputs=1
  Logical Operator1 : Logic  Operator=XOR
  Logical Operator3 : Logic
  Logical Operator4 : Logic
  MaxPeak : Subsystem
  Memory2 : Memory
  MinPeak : Subsystem
  Relational Operator : RelationalOperator  Operator=>  RndMeth=Nearest  InputSameDT=on
  Scope1 : Scope
  Sign : Signum
  Sum4 : Sum  InputSameDT=on  SaturateOnIntegerOverflow=on  OutDataTypeStr=Inherit: Same as first input
  Switch2 : Switch  Threshold=0.5  SaturateOnIntegerOverflow=on  InputSameDT=on
  Transfer Fcn1 : TransferFcn  Numerator=[1 0]  Denominator=[0.05 1]
  h : Gain  Gain=8  SaturateOnIntegerOverflow=on  OutDataTypeStr=Inherit: Same as input  ParamDataTypeStr=Inherit: Same as input
  MRFT Output : Outport  VectorParamsAs1DForOutWhenUnconnected=off
  wires:
  MaxPeak/1(Out) -> Display/1, Switch2/1
  Beta/1 -> Sum4/2
  Error/1 -> Gain5/1, Sum4/1, Gain4/1
  Gain5/1 -> Transfer Fcn1/1
  Memory2/1 -> Logical Operator1/2
  Logical Operator3/1 -> MinPeak/2(Cntrl)
  Relational Operator/1 -> Logical Operator/1, Logical Operator1/1, Memory2/1, Logical Operator3/2, Switch2/2
  Sign/1 -> h/1
  Transfer Fcn1/1 -> Relational Operator/1
  Constant4/1 -> Relational Operator/2
  Gain4/1 -> MinPeak/1(In), MaxPeak/2(In)
  Switch2/1 -> Beta/1
  Sum4/1 -> Sign/1
  Logical Operator/1 -> Logical Operator4/2
  Logical Operator1/1 -> Logical Operator4/1, Logical Operator3/1
  Logical Operator4/1 -> MaxPeak/1(Cntrl)
  h/1 -> MRFT Output/1, Scope1/1
  MinPeak/1(Out) -> Display1/1, Switch2/3

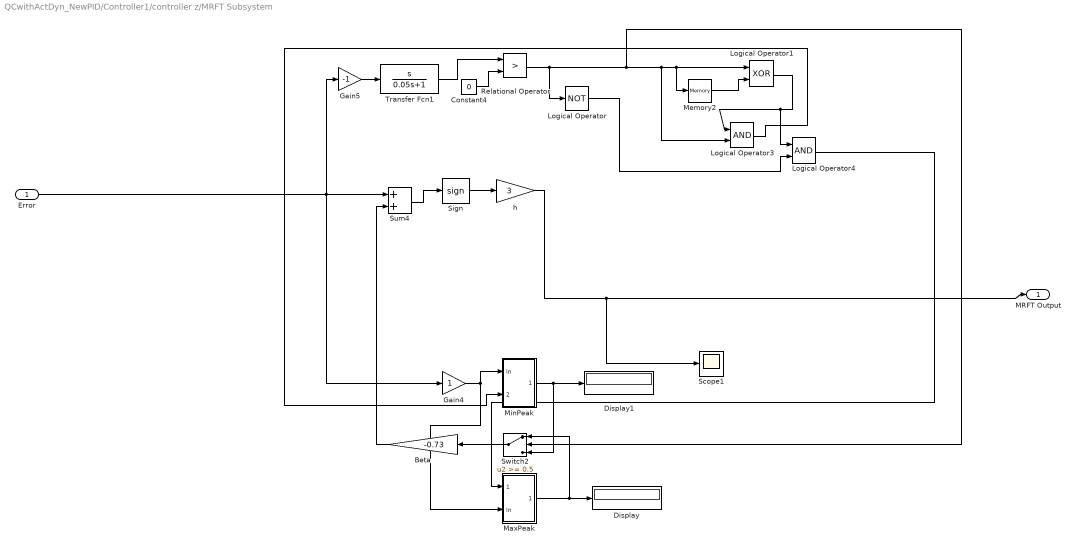
== system QCwithActDyn_NewPID/Controller1/controller z/MRFT Subsystem ==
  Error : Inport
  Beta : Gain  Gain=-0.73  SaturateOnIntegerOverflow=on  OutDataTypeStr=Inherit: Same as input  ParamDataTypeStr=Inherit: Same as input
  Constant4 : Constant  Value=0
  Display : Display
  Display1 : Display
  Gain4 : Gain  SaturateOnIntegerOverflow=on  OutDataTypeStr=Inherit: Same as input  ParamDataTypeStr=Inherit: Same as input
  Gain5 : Gain  Gain=-1  SaturateOnIntegerOverflow=on  OutDataTypeStr=Inherit: Same as input  ParamDataTypeStr=Inherit: Same as input
  Logical Operator : Logic  Operator=NOT  Inputs=1
  Logical Operator1 : Logic  Operator=XOR
  Logical Operator3 : Logic
  Logical Operator4 : Logic
  MaxPeak : Subsystem
  Memory2 : Memory
  MinPeak : Subsystem
  Relational Operator : RelationalOperator  Operator=>  RndMeth=Nearest  InputSameDT=on
  Scope1 : Scope
  Sign : Signum
  Sum4 : Sum  InputSameDT=on  SaturateOnIntegerOverflow=on  OutDataTypeStr=Inherit: Same as first input
  Switch2 : Switch  Threshold=0.5  SaturateOnIntegerOverflow=on  InputSameDT=on
  Transfer Fcn1 : TransferFcn  Numerator=[1 0]  Denominator=[0.05 1]
  h : Gain  Gain=3  SaturateOnIntegerOverflow=on  OutDataTypeStr=Inherit: Same as input  ParamDataTypeStr=Inherit: Same as input
  MRFT Output : Outport  VectorParamsAs1DForOutWhenUnconnected=off
  wires:
  MaxPeak/1(Out) -> Display/1, Switch2/1
  Beta/1 -> Sum4/2
  Error/1 -> Gain5/1, Sum4/1, Gain4/1
  Gain5/1 -> Transfer Fcn1/1
  Memory2/1 -> Logical Operator1/2
  Logical Operator3/1 -> MinPeak/2(Cntrl)
  Relational Operator/1 -> Logical Operator/1, Logical Operator1/1, Memory2/1, Logical Operator3/2, Switch2/2
  Sign/1 -> h/1
  Transfer Fcn1/1 -> Relational Operator/1
  Constant4/1 -> Relational Operator/2
  Gain4/1 -> MinPeak/1(In), MaxPeak/2(In)
  Switch2/1 -> Beta/1
  Sum4/1 -> Sign/1
  Logical Operator/1 -> Logical Operator4/2
  Logical Operator1/1 -> Logical Operator4/1, Logical Operator3/1
  Logical Operator4/1 -> MaxPeak/1(Cntrl)
  h/1 -> MRFT Output/1, Scope1/1
  MinPeak/1(Out) -> Display1/1, Switch2/3

== system QCwithActDyn_NewPID/Controller1/controller x/MRFT Subsystem/MaxPeak ==
  Cntrl : Inport
  In : Inport  Port=2
  Constant2 : Constant  Value=0
  Memory : Memory
  MinMax : MinMax  Function=max  Inputs=2  InputSameDT=on  SaturateOnIntegerOverflow=on
  Switch : Switch  Threshold=0.5  SaturateOnIntegerOverflow=on  InputSameDT=on
  Out : Outport  VectorParamsAs1DForOutWhenUnconnected=off
  wires:
  MinMax/1 -> Memory/1, Out/1
  Switch/1 -> MinMax/1
  Constant2/1 -> Switch/1
  Memory/1 -> Switch/3
  In/1 -> MinMax/2
  Cntrl/1 -> Switch/2

== system QCwithActDyn_NewPID/Controller1/controller x/MRFT Subsystem/MinPeak ==
  In : Inport
  Cntrl : Inport  Port=2
  Constant3 : Constant  Value=0
  Memory1 : Memory
  MinMax1 : MinMax  Inputs=2  InputSameDT=on  SaturateOnIntegerOverflow=on
  Switch1 : Switch  Threshold=0.5  SaturateOnIntegerOverflow=on  InputSameDT=on
  Out : Outport  VectorParamsAs1DForOutWhenUnconnected=off
  wires:
  MinMax1/1 -> Memory1/1, Out/1
  Switch1/1 -> MinMax1/2
  Memory1/1 -> Switch1/3
  Constant3/1 -> Switch1/1
  In/1 -> MinMax1/1
  Cntrl/1 -> Switch1/2

== system QCwithActDyn_NewPID/Controller1/controller z/MRFT Subsystem/MaxPeak ==
  Cntrl : Inport
  In : Inport  Port=2
  Constant2 : Constant  Value=0
  Memory : Memory
  MinMax : MinMax  Function=max  Inputs=2  InputSameDT=on  SaturateOnIntegerOverflow=on
  Switch : Switch  Threshold=0.5  SaturateOnIntegerOverflow=on  InputSameDT=on
  Out : Outport  VectorParamsAs1DForOutWhenUnconnected=off
  wires:
  MinMax/1 -> Memory/1, Out/1
  Switch/1 -> MinMax/1
  Constant2/1 -> Switch/1
  Memory/1 -> Switch/3
  In/1 -> MinMax/2
  Cntrl/1 -> Switch/2

== system QCwithActDyn_NewPID/Controller1/controller z/MRFT Subsystem/MinPeak ==
  In : Inport
  Cntrl : Inport  Port=2
  Constant3 : Constant  Value=0
  Memory1 : Memory
  MinMax1 : MinMax  Inputs=2  InputSameDT=on  SaturateOnIntegerOverflow=on
  Switch1 : Switch  Threshold=0.5  SaturateOnIntegerOverflow=on  InputSameDT=on
  Out : Outport  VectorParamsAs1DForOutWhenUnconnected=off
  wires:
  MinMax1/1 -> Memory1/1, Out/1
  Switch1/1 -> MinMax1/2
  Memory1/1 -> Switch1/3
  Constant3/1 -> Switch1/1
  In/1 -> MinMax1/1
  Cntrl/1 -> Switch1/2

== matlab function QCwithActDyn_NewPID/Controller1/DCM constructor 1 ==
  data: roll input; DCM output; pitch input; yaw input
function DCM = fcn(roll, pitch, yaw)

%DCM of yaw
yaw_DCM = [cos(yaw) -sin(yaw) 0;
            sin(yaw) cos(yaw) 0;
            0 0 1];
        
% pitch_DCM = [cos(pitch) 0 sin(pitch);
%             0, 1, 0;
%             -sin(pitch) 0 cos(pitch)];
%         
% roll_DCM = [1, 0, 0;
%             0 cos(yaw) -sin(roll);
%             0 sin(roll) cos(roll)];
%      
% DCM = yaw_DCM * pitch_DCM * roll_DCM;


% DCM of roll/pitch
theta_err = norm([roll, pitch, 0]);
euler_axis_err = [0, 0, 0];
if(theta_err ~= 0)
    euler_axis_err = [roll, pitch, 0] / theta_err;
end
%limit theta_ref
theta_err = min(pi/2, max(theta_err, -pi/2));
quaternion_err = euler_axis_err * sin(theta_err / 2);
quaternion_err = [cos(theta_err / 2), quaternion_err];
roll_pitch_DCM = quat2rotm(quaternion_err);


DCM = yaw_DCM * roll_pitch_DCM;

end

== matlab function QCwithActDyn_NewPID/Controller1/Rotation Matrix5/reference correction ==
  data: yaw input; x_out output; x input; y input; y_out output
function [x_out,y_out] = fcn(yaw, x, y)

dcm = [cos(yaw) sin(yaw); -sin(yaw) cos(yaw)];

out = dcm * [x; y];
x_out = out(1);
y_out = out(2);

== matlab function QCwithActDyn_NewPID/Subsystem/reference correction ==
  data: yaw input; x_out output; x input; y input; y_out output
function [x_out,y_out] = fcn(yaw, x, y)

dcm = [cos(yaw) sin(yaw); -sin(yaw) cos(yaw)];

out = dcm * [x; y];
x_out = out(1);
y_out = out(2);

== matlab function QCwithActDyn_NewPID/Subsystem/reference correction1 ==
  data: yaw input; x_out output; x input; y input; y_out output
function [x_out,y_out] = fcn(yaw, x, y)

dcm = [cos(yaw) sin(yaw); -sin(yaw) cos(yaw)];

out = dcm * [x; y];
x_out = out(1);
y_out = out(2);

== matlab function QCwithActDyn_NewPID/Subsystem/MATLAB Function1 ==
  settings: updateMethod=DISCRETE
  data: enable input; x output; time input; y output; z output; yaw output; xdot output; ydot output; zdot output; xddot output; yddot output; done output
function [x, y, z, yaw, xdot, ydot, zdot ,xddot , yddot, done]= fcn(enable, time)

persistent start_time
persistent poly_x
persistent poly_y
persistent poly_z
persistent n_order
persistent ts
persistent trajectory_segment
persistent state 
%states:
%   1: First trajectory
%   2: Second trajectory
%   3: Third trajectory


if isempty(start_time) || isempty(trajectory_segment) || ~enable || isempty(state)
    start_time = time;
    trajectory_segment = 1;
    state = 1;
end

if isempty(poly_x) || isempty(poly_y) || isempty(poly_z) || isempty(ts)
    g = coder.load('8shape_15s_1-5m');
    poly_t = g.x_solution;
    n_order = g.poly_order;
    ts = g.T;
end

T = 15;
time_scale = 15/8;
R = 1.5;
x = 0; y = 0; z = 1; yaw=0; done=false;
xdot = 0; ydot = 0; zdot = 0;
xddot = 0; yddot = 0;
if enable
    t = time - start_time;
    if t > (T/time_scale)
        x = 0; y = 0; z = 1; yaw = 0; done = true;
        xdot = 0; ydot = 0; zdot = 0;
        xddot = 0; yddot = 0;
        return;
    end
    
    ft = 0;
    fdt = 0;
    fddt = 0;
    
    for i=0:n_order-1
        ft = ft + poly_t(i+1) * (t*time_scale)^i;
        if i>0
        fdt = fdt + i * poly_t(i+1) * (t*time_scale)^(i-1) * (time_scale);
        end
        if i>1
        fddt = fddt + i*(i-1)* poly_t(i+1) * (t*time_scale)^(i-2) * (time_scale)^2;
        end
    end
    ft = 2*pi*ft/T - pi/2;
    fdt = 2*pi*fdt/T;
    fddt = 2*pi*fddt/T;

    x = R*0.5*sin(2*ft);
    y = R*cos(ft);
    
    xdot = R*cos(2*ft)*fdt;
    ydot = -R*sin(ft)*fdt;
    
    xddot = R*(-sin(2*ft)*2*fdt^2 + cos(2*ft)*fddt);
    yddot = -R*(cos(ft)*fdt^2 + sin(ft)*fddt);
    
end

% if isempty(poly_x) || isempty(poly_y) || isempty(poly_z) || isempty(ts)
%     g = coder.load('90_deg_roll24.mat');
%     poly_x = g.polys_x;
%     poly_y = g.polys_y;
%     poly_z = g.polys_z;
%     n_order = g.n_order(1);
%     ts = g.ts;
% end
% 
% x = -3; y = 0; z = 0.75; yaw=0; done=false;
% xdot = 0; ydot = 0; zdot = 0; 
% if enable
%     t = time - start_time;
%     if t > ts(end)
%         t=ts(end)
%     elseif t > ts(trajectory_segment + 1)
%         trajectory_segment = trajectory_segment + 1;
%     end
% 
% %     poly_x_i = poly_x(:, trajectory_segment);
% %     poly_y_i = poly_y(:, trajectory_segment);
% %     poly_z_i = poly_z(:, trajectory_segment);
%     poly_x_i = poly_x{trajectory_segment};
%     poly_y_i = poly_y{trajectory_segment};
%     poly_z_i = poly_z{trajectory_segment};
% 
%     x = 0; y = 0; z = 0.15;
%     for i=0:n_order
%         x = x + poly_x_i(i+1) * t^i;
%         y = y + poly_y_i(i+1) * t^i;
%         z = z + poly_z_i(i+1) * t^i;
%         if i>0
%             xdot = xdot + i * poly_x_i(i+1) * t^(i-1);
%             ydot = ydot + i * poly_y_i(i+1) * t^(i-1);
%             zdot = zdot + i * poly_z_i(i+1) * t^(i-1);
%         end
%     end
% end


% if isempty(poly_x) || isempty(poly_y) || isempty(poly_z) || isempty(n_order) || isempty(ts)
%     g = coder.load('90_deg_roll24.mat');
%     poly_x = g.polys_x;
%     poly_y = g.polys_y;
%     poly_z = g.polys_z;
%     n_order = g.n_order(1);
%     ts = g.ts;
% end
% 
% 
% x = -3; y = 0; z = 0.75; yaw=0; done=false;
% xdot = 0; ydot = 0; zdot = 0; 
% if enable
%     t = time - start_time; 
%     tt = t;
%     if t > ts(end)
%         tt = ts(end);
%     elseif t > ts(trajectory_segment + 1)
%         trajectory_segment = trajectory_segment + 1;
%     end
% 
%     poly_x_i = poly_x(:, trajectory_segment);
%     poly_y_i = poly_y(:, trajectory_segment);
%     poly_z_i = poly_z(:, trajectory_segment);
%     poly_x_i = poly_x{trajectory_segment};
%     poly_y_i = poly_y{trajectory_segment};
%     poly_z_i = poly_z{trajectory_segment};
% 
%     offset = [0, 0, 0];
%     if state == 1
%         offset = [0, 0, 0.15];
%     elseif state == 2
%         offset = [0, 0, 0.15];
%     elseif state == 3
%         offset = [-0.25, 0.2, 0.25];
%     end
%     x = offset(1); y = offset(2); z = offset(3);
%     for i=0:n_order
%         x = x + poly_x_i(i+1) * tt^i;
%         y = y + poly_y_i(i+1) * tt^i;
%         z = z + poly_z_i(i+1) * tt^i;
%         if i>0
%             xdot = xdot + i * poly_x_i(i+1) * tt^(i-1);
%             ydot = ydot + i * poly_y_i(i+1) * tt^(i-1);
%             zdot = zdot + i * poly_z_i(i+1) * tt^(i-1);
%         end
%     end
%     
%     if t > ts(end)+0.5
%         switch state
%             case 1
%                 state = 2;
%                 start_time = time;
%                 g = coder.load('reset_traj_24_16.mat');
%                 poly_x = g.polys_x;
%                 poly_y = g.polys_y;
%                 poly_z = g.polys_z;
%                 n_order = g.n_order(1);
%                 ts = g.ts;
%                 trajectory_segment = 1;
%             case 2
%                 if t > ts(end)+6
%                     state = 3;
%                     start_time = time;
%                     g = coder.load('90_deg_roll16.mat');                
%                     poly_x = g.polys_x;
%                     poly_y = g.polys_y;
%                     poly_z = g.polys_z;
%                     n_order = g.n_order(1);
%                     ts = g.ts;     
%                     trajectory_segment = 1;       
%                 end
%                 
%         end
%     end
        
% end

== matlab function QCwithActDyn_NewPID/Controller1/Thrust modulator ==
  data: input_thrust input; output_thrust output
function output_thrust = fcn(input_thrust)

output_thrust = input_thrust;
if max(input_thrust) > 1
    output_thrust = input_thrust - max(input_thrust) + 1;
elseif min(input_thrust) < 0.05
    output_thrust = input_thrust - min(input_thrust) + 0.05;
end

== matlab function QCwithActDyn_NewPID/Controller1/throttle limiter ==
  data: throttle_in input; e_roll input; e_pitch input; e_yaw input; throttle_out output
function throttle_out = fcn(throttle_in, e_roll, e_pitch, e_yaw)

throttle_out = throttle_in * cos(norm([e_roll, e_pitch, e_yaw]));

if (throttle_out < 0) 
    throttle_out = 0;
end

== matlab function QCwithActDyn_NewPID/Quadcopter Dynamics1/Nonlinear Dynamics/kinematic differential equation ==
  settings: updateMethod=DISCRETE
  data: roll_rate input; quat_rate output; pitch_rate input; yaw_rate input; t input; quat_in input; quat output; DCM output; roll output; pitch output; yaw output
function [quat_rate, quat, DCM, roll, pitch, yaw]  = fcn(roll_rate, pitch_rate, yaw_rate, t, quat_in)

persistent last_t;

if isempty(last_t)
    last_t = 0;
end


quat_tilde = [-quat_in(2), -quat_in(3), -quat_in(4);
            quat_in(1), -quat_in(4), quat_in(3);
            quat_in(4), quat_in(1), -quat_in(2);
            -quat_in(3), quat_in(2), quat_in(1)];

quat_rate = 0.5 * quat_tilde * [roll_rate; pitch_rate; yaw_rate];

quat_a = quat_in + quat_rate * (t-last_t);

quat_a = quat_a / norm(quat_a);

quat = quat_a';

q0 = quat(1); q1=quat(2); q2=quat(3); q3=quat(4);
DCM = [(q0^2 + q1^2 - q2^2 - q3^2), 2*(q1*q2+q0*q3), 2*(q1*q3-q0*q2);
        2*(q1*q2-q0*q3), (q0^2 - q1^2 + q2^2 - q3^2), 2*(q2*q3+q0*q1);
        2*(q1*q3+q0*q2), 2*(q2*q3-q0*q1), (q0^2 - q1^2 - q2^2 + q3^2)];

%yaw as euler angle
euler_angle = quat2eul(quat, 'ZYX');
yaw = euler_angle(1);

yaw_DCM = eul2rotm([0, 0, yaw], 'XYZ');

DCM_without_yaw = yaw_DCM' * DCM;
rotation_vector = rotationMatrixToVector(DCM_without_yaw);

%roll and pitch as rotation vectors
roll = rotation_vector(1); 
pitch = rotation_vector(2);


if(abs(pitch_rate)>0.1)
   roll_rate; 
end

DCM = DCM';
last_t = t;

== matlab function QCwithActDyn_NewPID/Subsystem/MATLAB Function ==
  settings: updateMethod=DISCRETE
  data: enable input; px output; time input; vx output; ax output; jx output; py output; vy output; ay output; jy output; t output; i output
function [px, vx, ax, jx, py, vy, ay, jy,t,i] = xy_pvaj(enable,time)

persistent start_time
persistent ts
persistent xvals
persistent yvals

if isempty(start_time) || ~enable
    start_time = time;
    g = coder.load('xy_tpvaj.mat');
    xvals = g.x_tpvaj;
    yvals = g.y_tpvaj;
    ts = xvals(1,end);
end

px = 0; vx = 0; ax = 0; jx = 0;
py = 0; vy = 0; ay = 0; jy = 0; t = 0; i = 0;

if enable
    t = time - start_time;
    
    if t > ts
        px = 0; vx = 0; ax = 0; jx = 0;
        py = 0; vy = 0; ay = 0; jy = 0; t = 0; i = 0;
        return;
    end
    
    i = round(t*(length(xvals)-1)/ts) + 1;
    if i == (length(xvals)-1)+1
        
        px = 0; vx = 0; ax = 0; jx = 0;
        py = 0; vy = 0; ay = 0; jy = 0; t = 0; i = 0;
        
    else
        
        px = xvals(2,i);
        vx = xvals(3,i);
        ax = xvals(4,i);
        jx = xvals(5,i);
        py = yvals(2,i);
        vy = yvals(3,i);
        ay = yvals(4,i);
        jy = yvals(5,i);
        
    end
end

end

== matlab function QCwithActDyn_NewPID/Controller1/attitude mapper  ==
  data: fx input; f output; fy input; fz input; roll_ref output; pitch_ref output
function [f, roll_ref, pitch_ref] = fcn(fx, fy, fz)

if fz>0
    f = sqrt(fx*fx + fy*fy + fz*fz);
else
    f = sqrt(fx*fx + fy*fy + 0);
end

unit_x_vector = [1, 0, 0];
unit_y_vector = [0, 1, 0];
unit_z_vector = [0, 0, 1];

if f == 0
    roll_ref = 0;
    pitch_ref = 0;    
else
    fz=abs(fz);
    force_vector = [fx, fy, fz];
    theta = acos(dot(unit_z_vector, force_vector) / norm(force_vector));
    
    if theta==0
        roll_ref = 0;
        pitch_ref = 0; 
    else        
        force_xy_projection = [fx; fy] / norm([fx; fy]);
        rotation_vector = [cos(pi/2) -sin(pi/2); sin(pi/2) cos(pi/2)] * force_xy_projection;
        roll_ref = theta * rotation_vector(1);
        pitch_ref = theta * rotation_vector(2);
    end
end

end

== matlab function QCwithActDyn_NewPID/Controller1/Rotation Matrix2/reference correction ==
  data: yaw input; x_out output; x input; y input; y_out output
function [x_out,y_out] = fcn(yaw, x, y)

dcm = [cos(yaw) sin(yaw); -sin(yaw) cos(yaw)];

out = dcm * [x; y];
x_out = out(1);
y_out = out(2);

== matlab function QCwithActDyn_NewPID/Controller1/Body frame attitude error1 ==
  data: roll_ref input; pitch_ref input; yaw_ref input; e_roll output; e_pitch output; e_yaw output; DCM input
function [e_roll, e_pitch, e_yaw] = fcn(roll_ref, pitch_ref, yaw_ref, DCM)

DCM_yaw_ref = [cos(yaw_ref), -sin(yaw_ref), 0;
                sin(yaw_ref), cos(yaw_ref), 0;
                0, 0, 1];

yaw_ref = 0;
theta_ref = norm([roll_ref, pitch_ref, yaw_ref]);

if(theta_ref ~= 0)
    euler_axis_ref = [roll_ref, pitch_ref, yaw_ref] / theta_ref;
else
    euler_axis_ref = [0, 0, 0];
end

%limit theta_ref
theta_ref = min(pi/2, max(theta_ref, -pi/2));

quaternion_ref = euler_axis_ref * sin(theta_ref / 2);
quaternion_ref = [cos(theta_ref / 2), quaternion_ref];

DCM_ref = DCM_yaw_ref * quat2rotm(quaternion_ref);

DCM_error = transpose(DCM) * DCM_ref;

g = trace((trace(DCM_error) - 1) / 2);
g = min(1, max(g, -1));
theta_error = acos(g);

if(theta_error ~= 0)
    e_roll = theta_error * ( DCM_error(3,2) - DCM_error(2,3) ) / (2 * sin(theta_error));
    e_pitch = theta_error * ( DCM_error(1,3) - DCM_error(3,1) ) / (2 * sin(theta_error));
    e_yaw = theta_error * ( DCM_error(2,1) - DCM_error(1,2) ) / (2 * sin(theta_error));
else
    e_roll = 0;
    e_pitch = 0;
    e_yaw = 0;
end


end

== matlab function QCwithActDyn_NewPID/Controller1/Rotation Matrix3/reference correction ==
  data: yaw input; x_out output; x input; y input; y_out output
function [x_out,y_out] = fcn(yaw, x, y)

dcm = [cos(yaw) sin(yaw); -sin(yaw) cos(yaw)];

out = dcm * [x; y];
x_out = out(1);
y_out = out(2);

== matlab function QCwithActDyn_NewPID/Controller1/Rotation Matrix4/reference correction ==
  data: yaw input; x_out output; x input; y input; y_out output
function [x_out,y_out] = fcn(yaw, x, y)

dcm = [cos(yaw) sin(yaw); -sin(yaw) cos(yaw)];

out = dcm * [x; y];
x_out = out(1);
y_out = out(2);
